simulink model "ResearchPaper3Fig3"  (R2015b)
settings: Solver=VariableStepAuto  StartTime=0.0  StopTime=10.0  RelTol=1e-3
libraries: xbsIndex_r4 x544, commfilt2 x1, commrandsrc3 x1, commdigbbndam3 x1
(part 1 of 4)
settings Model: Creator=barna  LastModifiedBy=barna

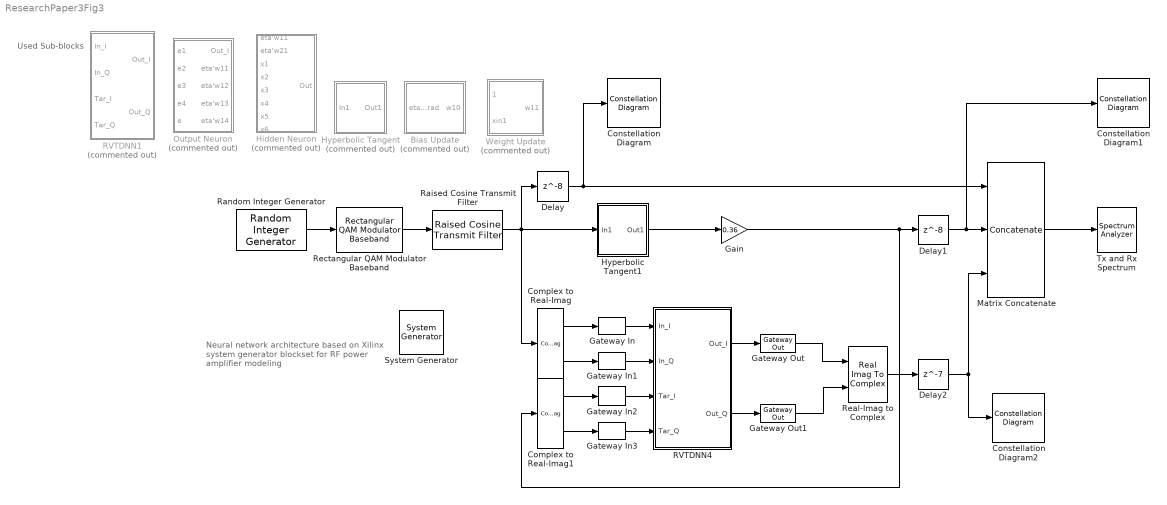
== system ResearchPaper3Fig3 ==
  note: Neural network architecture based on Xilinx system generator blockset for RF power amplifier modeling
  note: Used Sub-blocks
  " System Generator" : xbsIndex_r4/ System Generator  Tag=genX  xilinxfamily=kintex7  part=xc7k325t  speed=-3  package=fbg676  synthesis_tool=Vivado  clock_wrapper=Clock Enables  directory=./netlist  proj_type=Vivado  Synth_file=Vivado Synthesis Defaults  Impl_file=Vivado Implementation Defaults  testbench=off  simulink_period=1  sysclk_period=10  dcm_input_clock_period=10  incr_netlist=off  trim_vbits=Everywhere in SubSystem  dbl_ovrd=According to Block Masks  core_generation=According to Block Masks  run_coregen=off  deprecated_control=off  eval_field=0  block_type=sysgen
  Bias Update : Subsystem  Commented=on
  Complex to Real-Imag : ComplexToRealImag
  Complex to Real-Imag1 : ComplexToRealImag
  Constellation Diagram : ConstellationDiagram
  Constellation Diagram1 : ConstellationDiagram
  Constellation Diagram2 : ConstellationDiagram
  Delay : Delay  DelayLength=8  InitialCondition=0
  Delay1 : Delay  DelayLength=8  InitialCondition=0
  Delay2 : Delay  DelayLength=7  InitialCondition=0
  Gain : Gain  Gain=0.36
  Gateway In{,1..3} (4 alike) : xbsIndex_r4/Gateway In  gui_display_data_type=Fixed-point  arith_type="Signed  (2's comp)"  n_bits=16  bin_pt=14  preci_type=Single  exp_width=8  frac_width=24  rows=1  columns=1  quantization="Round  (unbiased: +/- Inf)"  overflow=Saturate  period=1  UseAsADC=off  ADCChannel='1'  interface=None  automatic_assignment=on  address_offset=hex2dec('00')  intf_name=''  intf_description=''  default_value=0  timing_constraint=None  locs_specified=off  LOCs={}  io_standard={}  inherit_from_input=off  hdl_port=on  dbl_ovrd=off  block_type=gatewayin
  Gateway Out : xbsIndex_r4/Gateway Out  inherit_from_input=off  hdl_port=on  rows=1  columns=1  UseAsDAC=off  DACChannel='1'  interface=None  automatic_assignment=on  address_offset=hex2dec('00')  intf_name=''  intf_description=''  timing_constraint=None  locs_specified=off  LOCs={}  io_standard={}  block_type=gatewayout
  Gateway Out1 : xbsIndex_r4/Gateway Out  inherit_from_input=off  hdl_port=on  rows=1  columns=1  UseAsDAC=off  DACChannel='1'  interface=None  automatic_assignment=on  address_offset=hex2dec('00')  intf_name=''  intf_description=''  timing_constraint=None  locs_specified=off  LOCs={}  io_standard={}  block_type=gatewayout
  Hidden Neuron : Subsystem  Commented=on
  Hyperbolic Tangent : Subsystem  Commented=on
  Hyperbolic Tangent1 : Subsystem
  Matrix Concatenate : Concatenate  NumInputs=3  Mode=Multidimensional array  ConcatenateDimension=2
  Output Neuron : Subsystem  Commented=on
  RVTDNN1 : Subsystem  Commented=on
  RVTDNN4 : Subsystem
  Raised Cosine Transmit Filter : commfilt2/Raised Cosine Transmit Filter  filtType=Normal  filtSpan=20  currentFiltSpan=20  D=(20)/2  R=0.2  sampMode=Mute  saveAsFlag=0  N=20  framing=Enforce single-rate processing  InputProcessing=Columns as channels (frame based)  checkGain=Normalized  filterGain=1  checkCoeff=off  variableName=rcTxFilt  launchFVT=on  roundingMode=Floor  overflowMode=off
  Random Integer Generator : commrandsrc3/Random Integer Generator  SetSize=8  SeedSource=Auto  Seed=0  SampleTime=1  SamplesPerFrame=1  OutputDataType=double  SimulateUsing=Interpreted execution
  Real-Imag to Complex : RealImagToComplex
  Rectangular QAM Modulator Baseband : commdigbbndam3/Rectangular QAM Modulator Baseband  M=16  InType=Integer  Enc=Gray  Mapping=[0:15]  PowType=Min. distance between symbols  MinDist=2  AvgPow=1  PeakPow=1  Ph=0  outDtype=double  outWordLen=16  outUDDataType=sfix(16)  outFracLenMode=Best precision  outFracLen=15
  Tx and Rx Spectrum : SpectrumAnalyzer
  Weight Update : Subsystem  Commented=on
  wires:
  Random Integer Generator/1 -> Rectangular QAM Modulator Baseband/1
  Rectangular QAM Modulator Baseband/1 -> Raised Cosine Transmit Filter/1
  Raised Cosine Transmit Filter/1 -> Hyperbolic Tangent1/1(In1), Complex to Real-Imag/1, Delay/1
  Complex to Real-Imag/1 -> Gateway In/1
  Complex to Real-Imag/2 -> Gateway In1/1
  Complex to Real-Imag1/1 -> Gateway In2/1
  Complex to Real-Imag1/2 -> Gateway In3/1
  Gateway Out/1 -> Real-Imag to Complex/1
  Gateway Out1/1 -> Real-Imag to Complex/2
  Gain/1 -> Complex to Real-Imag1/1, Delay1/1
  Real-Imag to Complex/1 -> Delay2/1
  Delay1/1 -> Constellation Diagram1/1, Matrix Concatenate/2
  Delay/1 -> Constellation Diagram/1, Matrix Concatenate/1
  Delay2/1 -> Matrix Concatenate/3, Constellation Diagram2/1
  Matrix Concatenate/1 -> Tx and Rx Spectrum/1
  Gateway In/1 -> RVTDNN4/1(In_I)
  Gateway In1/1 -> RVTDNN4/2(In_Q)
  Gateway In2/1 -> RVTDNN4/3(Tar_I)
  Gateway In3/1 -> RVTDNN4/4(Tar_Q)
  RVTDNN4/2(Out_Q) -> Gateway Out1/1
  RVTDNN4/1(Out_I) -> Gateway Out/1
  Hyperbolic Tangent1/1(Out1) -> Gain/1

== system ResearchPaper3Fig3/Bias Update ==
  eta'grad : Inport
  AddSub : xbsIndex_r4/AddSub  mode=Addition  use_carryin=off  use_carryout=off  en=off  latency=0  precision=Full  arith_type=Unsigned  n_bits=16  bin_pt=14  quantization=Truncate  overflow=Wrap  use_behavioral_HDL=off  hw_selection=Fabric  pipelined=off  dbl_ovrd=off  block_type=addsub
  Register : xbsIndex_r4/Register  init=0  rst=off  en=off  dbl_ovrd=off  block_type=register
  w10 : Outport
  wires:
  Register/1 -> w10/1, AddSub/2
  AddSub/1 -> Register/1
  eta'grad/1 -> AddSub/1

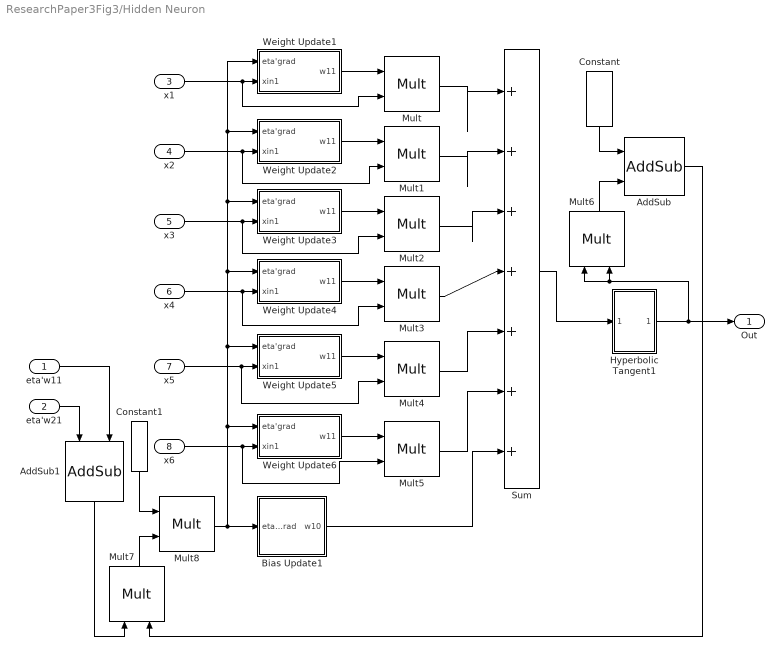
== system ResearchPaper3Fig3/Hidden Neuron ==
  eta'w11 : Inport
  eta'w21 : Inport  Port=2
  x1 : Inport  Port=3
  x2 : Inport  Port=4
  x3 : Inport  Port=5
  x4 : Inport  Port=6
  x5 : Inport  Port=7
  x6 : Inport  Port=8
  AddSub : xbsIndex_r4/AddSub  mode=Subtraction  use_carryin=off  use_carryout=off  en=off  latency=0  precision=Full  arith_type=Unsigned  n_bits=16  bin_pt=14  quantization=Truncate  overflow=Wrap  use_behavioral_HDL=off  hw_selection=Fabric  pipelined=off  dbl_ovrd=off  block_type=addsub
  AddSub1 : xbsIndex_r4/AddSub  mode=Addition  use_carryin=off  use_carryout=off  en=off  latency=0  precision=Full  arith_type=Unsigned  n_bits=16  bin_pt=14  quantization=Truncate  overflow=Wrap  use_behavioral_HDL=off  hw_selection=Fabric  pipelined=off  dbl_ovrd=off  block_type=addsub
  Bias Update1 : Subsystem
  Constant : xbsIndex_r4/Constant  const=1.0  gui_display_data_type=Fixed-point  arith_type=Signed (2's comp)  n_bits=16  bin_pt=14  preci_type=Single  exp_width=8  frac_width=24  explicit_period=off  period=1  equ=P=C  opselect=C  inp2=PCIN>>17  opr=+  inp1=P  carry=CIN  dbl_ovrd=off  block_type=constant
  Constant1 : xbsIndex_r4/Constant  const=0.1000000  gui_display_data_type=Fixed-point  arith_type=Signed (2's comp)  n_bits=32  bin_pt=24  preci_type=Single  exp_width=8  frac_width=24  explicit_period=off  period=1  equ=P=C  opselect=C  inp2=PCIN>>17  opr=+  inp1=P  carry=CIN  dbl_ovrd=off  block_type=constant
  Hyperbolic Tangent1 : Subsystem
  Mult{,1..8} (9 alike) : xbsIndex_r4/Mult  precision=Full  arith_type="Signed  (2's comp)"  n_bits=16  bin_pt=14  quantization=Truncate  overflow=Wrap  en=off  latency=0  use_behavioral_HDL=off  opt=Speed  use_embedded=on  optimum_pipeline=off  pipeline=on  dbl_ovrd=off  use_rpm=on  placement_style=Triangular  block_type=mult
  Sum : Sum  Inputs=|+++++++
  Weight Update1 : Subsystem
  Weight Update2 : Subsystem
  Weight Update3 : Subsystem
  Weight Update4 : Subsystem
  Weight Update5 : Subsystem
  Weight Update6 : Subsystem
  Out : Outport
  wires:
  Mult7/1 -> Mult8/2
  Sum/1 -> Hyperbolic Tangent1/1(In1)
  Bias Update1/1(w10) -> Sum/7
  Constant/1 -> AddSub/1
  Mult8/1 -> Weight Update6/1(eta'grad), Weight Update5/1(eta'grad), Weight Update4/1(eta'grad), Weight Update3/1(eta'grad), Weight Update2/1(eta'grad), Weight Update1/1(eta'grad), Bias Update1/1(eta'grad)
  Constant1/1 -> Mult8/1
  Mult6/1 -> AddSub/2
  eta'w11/1 -> AddSub1/2
  Hyperbolic Tangent1/1(Out1) -> Out/1, Mult6/1, Mult6/2
  AddSub1/1 -> Mult7/1
  AddSub/1 -> Mult7/2
  eta'w21/1 -> AddSub1/1
  Weight Update5/1(w11) -> Mult4/1
  x3/1 -> Mult2/2, Weight Update3/2(xin1)
  x5/1 -> Mult4/2, Weight Update5/2(xin1)
  Weight Update6/1(w11) -> Mult5/1
  Weight Update4/1(w11) -> Mult3/1
  x2/1 -> Mult1/2, Weight Update2/2(xin1)
  Weight Update1/1(w11) -> Mult/1
  Weight Update2/1(w11) -> Mult1/1
  Weight Update3/1(w11) -> Mult2/1
  x1/1 -> Mult/2, Weight Update1/2(xin1)
  x4/1 -> Mult3/2, Weight Update4/2(xin1)
  Mult1/1 -> Sum/2
  Mult4/1 -> Sum/5
  x6/1 -> Mult5/2, Weight Update6/2(xin1)
  Mult3/1 -> Sum/4
  Mult5/1 -> Sum/6
  Mult/1 -> Sum/1
  Mult2/1 -> Sum/3

== system ResearchPaper3Fig3/Hyperbolic Tangent ==
  In1 : Inport
  CMult : xbsIndex_r4/CMult  const=16380  gui_display_data_type=Fixed-point  const_n_bits=32  const_bin_pt=14  float_type=Single  exp_bits=8  fraction_bits=24  en=off  latency=0  precision=Full  arith_type="Signed  (2's comp)"  n_bits=16  bin_pt=14  quantization=Truncate  overflow=Wrap  use_behavioral_HDL=off  mem_type=Distributed RAM  pipeline=off  dbl_ovrd=off  block_type=cmult
  Constant : xbsIndex_r4/Constant  const=0.0  gui_display_data_type=Fixed-point  arith_type=Signed (2's comp)  n_bits=16  bin_pt=14  preci_type=Single  exp_width=8  frac_width=24  explicit_period=off  period=1  equ=P=C  opselect=C  inp2=PCIN>>17  opr=+  inp1=P  carry=CIN  dbl_ovrd=off  block_type=constant
  Delay1 : xbsIndex_r4/Delay  rst=off  infoeditControl=Selection of Reset will increase slice count due to use of real FFs and instead of SRLs  en=off  latency=1  reg_retiming=off  dbl_ovrd=off  block_type=delay
  Mux : xbsIndex_r4/Mux  inputs=2  en=off  latency=0  precision=Full  arith_type=Unsigned  n_bits=16  bin_pt=14  quantization=Truncate  overflow=Wrap  dbl_ovrd=off  block_type=mux
  Mux1 : xbsIndex_r4/Mux  inputs=2  en=off  latency=0  precision=Full  arith_type=Unsigned  n_bits=16  bin_pt=14  quantization=Truncate  overflow=Wrap  dbl_ovrd=off  block_type=mux
  Negate : xbsIndex_r4/Negate  precision=Full  arith_type=Unsigned  n_bits=16  bin_pt=14  quantization=Truncate  overflow=Wrap  en=off  latency=0  dbl_ovrd=off  block_type=negate
  Negate1 : xbsIndex_r4/Negate  precision=Full  arith_type=Unsigned  n_bits=16  bin_pt=14  quantization=Truncate  overflow=Wrap  en=off  latency=0  dbl_ovrd=off  block_type=negate
  ROM : xbsIndex_r4/ROM  depth=16  initVector=sin(pi*(0:15)/16)  distributed_mem=Block RAM  rst=off  init_reg=0  en=off  latency=1  gui_display_data_type=Fixed-point  arith_type="Signed  (2's comp)"  n_bits=16  bin_pt=14  preci_type=Single  exp_width=8  frac_width=24  optimize=Area  use_rpm=on  dbl_ovrd=off  block_type=sprom
  Relational : xbsIndex_r4/Relational  mode=a>b  op_type=Bool  en=off  latency=0  dbl_ovrd=off  block_type=relational
  Out1 : Outport
  wires:
  Delay1/1 -> Mux1/1
  Mux/1 -> CMult/1
  Mux1/1 -> Out1/1
  ROM/1 -> Negate1/1, Mux1/2
  Negate1/1 -> Mux1/3
  Relational/1 -> Delay1/1, Mux/1
  Constant/1 -> Relational/1
  In1/1 -> Negate/1, Relational/2, Mux/2
  Negate/1 -> Mux/3
  CMult/1 -> ROM/1

== system ResearchPaper3Fig3/Hyperbolic Tangent1 ==
  In1 : Inport
  CMult : xbsIndex_r4/CMult  const=16380  gui_display_data_type=Fixed-point  const_n_bits=32  const_bin_pt=14  float_type=Single  exp_bits=8  fraction_bits=24  en=off  latency=0  precision=Full  arith_type="Signed  (2's comp)"  n_bits=16  bin_pt=14  quantization=Truncate  overflow=Wrap  use_behavioral_HDL=off  mem_type=Distributed RAM  pipeline=off  dbl_ovrd=off  block_type=cmult
  Constant : xbsIndex_r4/Constant  const=0.0  gui_display_data_type=Fixed-point  arith_type=Signed (2's comp)  n_bits=16  bin_pt=14  preci_type=Single  exp_width=8  frac_width=24  explicit_period=off  period=1  equ=P=C  opselect=C  inp2=PCIN>>17  opr=+  inp1=P  carry=CIN  dbl_ovrd=off  block_type=constant
  Delay1 : xbsIndex_r4/Delay  rst=off  infoeditControl=Selection of Reset will increase slice count due to use of real FFs and instead of SRLs  en=off  latency=1  reg_retiming=off  dbl_ovrd=off  block_type=delay
  Mux : xbsIndex_r4/Mux  inputs=2  en=off  latency=0  precision=Full  arith_type=Unsigned  n_bits=16  bin_pt=14  quantization=Truncate  overflow=Wrap  dbl_ovrd=off  block_type=mux
  Mux1 : xbsIndex_r4/Mux  inputs=2  en=off  latency=0  precision=Full  arith_type=Unsigned  n_bits=16  bin_pt=14  quantization=Truncate  overflow=Wrap  dbl_ovrd=off  block_type=mux
  Negate : xbsIndex_r4/Negate  precision=Full  arith_type=Unsigned  n_bits=16  bin_pt=14  quantization=Truncate  overflow=Wrap  en=off  latency=0  dbl_ovrd=off  block_type=negate
  Negate1 : xbsIndex_r4/Negate  precision=Full  arith_type=Unsigned  n_bits=16  bin_pt=14  quantization=Truncate  overflow=Wrap  en=off  latency=0  dbl_ovrd=off  block_type=negate
  ROM : xbsIndex_r4/ROM  depth=16  initVector=sin(pi*(0:15)/16)  distributed_mem=Block RAM  rst=off  init_reg=0  en=off  latency=1  gui_display_data_type=Fixed-point  arith_type="Signed  (2's comp)"  n_bits=16  bin_pt=14  preci_type=Single  exp_width=8  frac_width=24  optimize=Area  use_rpm=on  dbl_ovrd=off  block_type=sprom
  Relational : xbsIndex_r4/Relational  mode=a>b  op_type=Bool  en=off  latency=0  dbl_ovrd=off  block_type=relational
  Out1 : Outport
  wires:
  Delay1/1 -> Mux1/1
  Mux/1 -> CMult/1
  Mux1/1 -> Out1/1
  ROM/1 -> Negate1/1, Mux1/2
  Negate1/1 -> Mux1/3
  Relational/1 -> Delay1/1, Mux/1
  Constant/1 -> Relational/1
  In1/1 -> Negate/1, Relational/2, Mux/2
  Negate/1 -> Mux/3
  CMult/1 -> ROM/1

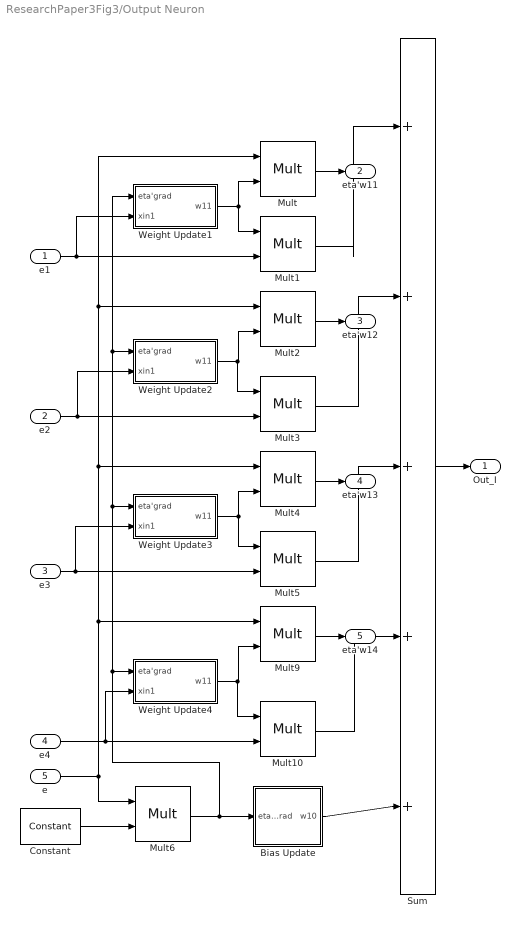
== system ResearchPaper3Fig3/Output Neuron ==
  e1 : Inport
  e2 : Inport  Port=2
  e3 : Inport  Port=3
  e4 : Inport  Port=4
  e : Inport  Port=5
  Bias Update : Subsystem
  Constant : xbsIndex_r4/Constant  const=16972656  gui_display_data_type=Fixed-point  arith_type=Signed (2's comp)  n_bits=64  bin_pt=14  preci_type=Single  exp_width=8  frac_width=24  explicit_period=off  period=1  equ=P=C  opselect=C  inp2=PCIN>>17  opr=+  inp1=P  carry=CIN  dbl_ovrd=off  block_type=constant
  Mult{,1..6,9..10} (9 alike) : xbsIndex_r4/Mult  precision=Full  arith_type="Signed  (2's comp)"  n_bits=16  bin_pt=14  quantization=Truncate  overflow=Wrap  en=off  latency=0  use_behavioral_HDL=off  opt=Speed  use_embedded=on  optimum_pipeline=off  pipeline=on  dbl_ovrd=off  use_rpm=on  placement_style=Triangular  block_type=mult
  Sum : Sum  Inputs=|+++++
  Weight Update1 : Subsystem
  Weight Update2 : Subsystem
  Weight Update3 : Subsystem
  Weight Update4 : Subsystem
  Out_I : Outport
  eta'w11 : Outport  Port=2
  eta'w12 : Outport  Port=3
  eta'w13 : Outport  Port=4
  eta'w14 : Outport  Port=5
  wires:
  e3/1 -> Weight Update3/2(xin1), Mult5/2
  e2/1 -> Weight Update2/2(xin1), Mult3/2
  e1/1 -> Weight Update1/2(xin1), Mult1/2
  e4/1 -> Weight Update4/2(xin1), Mult10/2
  Weight Update1/1(w11) -> Mult1/1, Mult/2
  Weight Update2/1(w11) -> Mult3/1, Mult2/2
  Weight Update3/1(w11) -> Mult5/1, Mult4/2
  Weight Update4/1(w11) -> Mult10/1, Mult9/2
  Mult/1 -> eta'w11/1
  Mult2/1 -> eta'w12/1
  Mult4/1 -> eta'w13/1
  Mult9/1 -> eta'w14/1
  Mult1/1 -> Sum/1
  Mult3/1 -> Sum/2
  Mult5/1 -> Sum/3
  Mult10/1 -> Sum/4
  Bias Update/1(w10) -> Sum/5
  Mult6/1 -> Weight Update4/1(eta'grad), Weight Update3/1(eta'grad), Weight Update2/1(eta'grad), Weight Update1/1(eta'grad), Bias Update/1(eta'grad)
  Constant/1 -> Mult6/2
  e/1 -> Mult4/1, Mult2/1, Mult/1, Mult9/1, Mult6/1
  Sum/1 -> Out_I/1

== system ResearchPaper3Fig3/RVTDNN1 ==
  In_I : Inport
  In_Q : Inport  Port=2
  Tar_I : Inport  Port=3
  Tar_Q : Inport  Port=4
  AddSub : xbsIndex_r4/AddSub  mode=Subtraction  use_carryin=off  use_carryout=off  en=off  latency=1  precision=Full  arith_type=Unsigned  n_bits=16  bin_pt=14  quantization=Truncate  overflow=Wrap  use_behavioral_HDL=off  hw_selection=Fabric  pipelined=off  dbl_ovrd=off  block_type=addsub
  AddSub1 : xbsIndex_r4/AddSub  mode=Subtraction  use_carryin=off  use_carryout=off  en=off  latency=1  precision=Full  arith_type=Unsigned  n_bits=16  bin_pt=14  quantization=Truncate  overflow=Wrap  use_behavioral_HDL=off  hw_selection=Fabric  pipelined=off  dbl_ovrd=off  block_type=addsub
  Delay{3..8} (6 alike) : xbsIndex_r4/Delay  rst=off  infoeditControl=Selection of Reset will increase slice count due to use of real FFs and instead of SRLs  en=off  latency=1  reg_retiming=off  dbl_ovrd=off  block_type=delay
  Hidden Neuron1 : Subsystem
  Hidden Neuron2 : Subsystem
  Hidden Neuron3 : Subsystem
  Hidden Neuron4 : Subsystem
  Output Neuron1 : Subsystem
  Output Neuron2 : Subsystem
  Out_I : Outport
  Out_Q : Outport  Port=2
  wires:
  Output Neuron2/1(Out_I) -> Out_Q/1, AddSub1/2
  Delay7/1 -> AddSub/1
  Output Neuron1/2(eta'w11) -> Hidden Neuron1/1(eta'w11)
  Delay8/1 -> AddSub1/1
  In_Q/1 -> Hidden Neuron3/6(x4), Hidden Neuron4/6(x4), Hidden Neuron1/6(x4), Hidden Neuron2/6(x4), Delay5/1
  Delay5/1 -> Hidden Neuron1/7(x5), Hidden Neuron2/7(x5), Hidden Neuron3/7(x5), Hidden Neuron4/7(x5), Delay6/1
  Delay3/1 -> Hidden Neuron2/4(x2), Hidden Neuron3/4(x2), Hidden Neuron4/4(x2), Hidden Neuron1/4(x2), Delay4/1
  Output Neuron2/3(eta'w12) -> Hidden Neuron2/2(eta'w21)
  Output Neuron2/4(eta'w13) -> Hidden Neuron3/2(eta'w21)
  AddSub/1 -> Output Neuron1/5(e)
  In_I/1 -> Hidden Neuron1/3(x1), Hidden Neuron2/3(x1), Hidden Neuron3/3(x1), Hidden Neuron4/3(x1), Delay3/1
  Output Neuron2/5(eta'w14) -> Hidden Neuron4/2(eta'w21)
  Hidden Neuron1/1(Out) -> Output Neuron2/1(e1), Output Neuron1/1(e1)
  Hidden Neuron4/1(Out) -> Output Neuron2/4(e4), Output Neuron1/4(e4)
  Hidden Neuron3/1(Out) -> Output Neuron2/3(e3), Output Neuron1/3(e3)
  Hidden Neuron2/1(Out) -> Output Neuron2/2(e2), Output Neuron1/2(e2)
  Output Neuron1/3(eta'w12) -> Hidden Neuron2/1(eta'w11)
  Output Neuron1/4(eta'w13) -> Hidden Neuron3/1(eta'w11)
  Output Neuron1/5(eta'w14) -> Hidden Neuron4/1(eta'w11)
  Output Neuron2/2(eta'w11) -> Hidden Neuron1/2(eta'w21)
  Delay6/1 -> Hidden Neuron1/8(x6), Hidden Neuron2/8(x6), Hidden Neuron3/8(x6), Hidden Neuron4/8(x6)
  Delay4/1 -> Hidden Neuron3/5(x3), Hidden Neuron4/5(x3), Hidden Neuron1/5(x3), Hidden Neuron2/5(x3)
  Tar_Q/1 -> Delay8/1
  Tar_I/1 -> Delay7/1
  AddSub1/1 -> Output Neuron2/5(e)
  Output Neuron1/1(Out_I) -> Out_I/1, AddSub/2

== system ResearchPaper3Fig3/RVTDNN4 ==
  In_I : Inport
  In_Q : Inport  Port=2
  Tar_I : Inport  Port=3
  Tar_Q : Inport  Port=4
  AddSub : xbsIndex_r4/AddSub  mode=Subtraction  use_carryin=off  use_carryout=off  en=off  latency=0  precision=Full  arith_type=Unsigned  n_bits=16  bin_pt=14  quantization=Truncate  overflow=Wrap  use_behavioral_HDL=off  hw_selection=Fabric  pipelined=off  dbl_ovrd=off  block_type=addsub
  AddSub1 : xbsIndex_r4/AddSub  mode=Subtraction  use_carryin=off  use_carryout=off  en=off  latency=0  precision=Full  arith_type=Unsigned  n_bits=16  bin_pt=14  quantization=Truncate  overflow=Wrap  use_behavioral_HDL=off  hw_selection=Fabric  pipelined=off  dbl_ovrd=off  block_type=addsub
  Delay{3..8} (6 alike) : xbsIndex_r4/Delay  rst=off  infoeditControl=Selection of Reset will increase slice count due to use of real FFs and instead of SRLs  en=off  latency=1  reg_retiming=off  dbl_ovrd=off  block_type=delay
  Hidden Neuron1 : Subsystem
  Hidden Neuron2 : Subsystem
  Hidden Neuron3 : Subsystem
  Hidden Neuron4 : Subsystem
  Output Neuron1 : Subsystem
  Output Neuron2 : Subsystem
  Out_I : Outport
  Out_Q : Outport  Port=2
  wires:
  Output Neuron2/1(Out_I) -> Out_Q/1, AddSub1/2
  Delay7/1 -> AddSub/1
  Output Neuron1/2(eta'w11) -> Hidden Neuron1/1(eta'w11)
  Delay8/1 -> AddSub1/1
  In_Q/1 -> Hidden Neuron3/6(x4), Hidden Neuron4/6(x4), Hidden Neuron1/6(x4), Hidden Neuron2/6(x4), Delay5/1
  Delay5/1 -> Hidden Neuron1/7(x5), Hidden Neuron2/7(x5), Hidden Neuron3/7(x5), Hidden Neuron4/7(x5), Delay6/1
  Delay3/1 -> Hidden Neuron2/4(x2), Hidden Neuron3/4(x2), Hidden Neuron4/4(x2), Hidden Neuron1/4(x2), Delay4/1
  Output Neuron2/3(eta'w12) -> Hidden Neuron2/2(eta'w21)
  Output Neuron2/4(eta'w13) -> Hidden Neuron3/2(eta'w21)
  AddSub/1 -> Output Neuron1/5(e)
  In_I/1 -> Hidden Neuron1/3(x1), Hidden Neuron2/3(x1), Hidden Neuron3/3(x1), Hidden Neuron4/3(x1), Delay3/1
  Output Neuron2/5(eta'w14) -> Hidden Neuron4/2(eta'w21)
  Hidden Neuron1/1(Out) -> Output Neuron2/1(e1), Output Neuron1/1(e1)
  Hidden Neuron4/1(Out) -> Output Neuron2/4(e4), Output Neuron1/4(e4)
  Hidden Neuron3/1(Out) -> Output Neuron2/3(e3), Output Neuron1/3(e3)
  Hidden Neuron2/1(Out) -> Output Neuron2/2(e2), Output Neuron1/2(e2)
  Output Neuron1/3(eta'w12) -> Hidden Neuron2/1(eta'w11)
  Output Neuron1/4(eta'w13) -> Hidden Neuron3/1(eta'w11)
  Output Neuron1/5(eta'w14) -> Hidden Neuron4/1(eta'w11)
  Output Neuron2/2(eta'w11) -> Hidden Neuron1/2(eta'w21)
  Delay6/1 -> Hidden Neuron1/8(x6), Hidden Neuron2/8(x6), Hidden Neuron3/8(x6), Hidden Neuron4/8(x6)
  Delay4/1 -> Hidden Neuron3/5(x3), Hidden Neuron4/5(x3), Hidden Neuron1/5(x3), Hidden Neuron2/5(x3)
  Tar_Q/1 -> Delay8/1
  Tar_I/1 -> Delay7/1
  AddSub1/1 -> Output Neuron2/5(e)
  Output Neuron1/1(Out_I) -> Out_I/1, AddSub/2

== system ResearchPaper3Fig3/Weight Update ==
  eta'grad : Inport
  xin1 : Inport  Port=2
  AddSub : xbsIndex_r4/AddSub  mode=Addition  use_carryin=off  use_carryout=off  en=off  latency=0  precision=Full  arith_type=Unsigned  n_bits=16  bin_pt=14  quantization=Truncate  overflow=Wrap  use_behavioral_HDL=off  hw_selection=Fabric  pipelined=off  dbl_ovrd=off  block_type=addsub
  Mult : xbsIndex_r4/Mult  precision=Full  arith_type="Signed  (2's comp)"  n_bits=16  bin_pt=14  quantization=Truncate  overflow=Wrap  en=off  latency=0  use_behavioral_HDL=off  opt=Speed  use_embedded=on  optimum_pipeline=off  pipeline=on  dbl_ovrd=off  use_rpm=on  placement_style=Triangular  block_type=mult
  Register : xbsIndex_r4/Register  init=0  rst=off  en=off  dbl_ovrd=off  block_type=register
  w11 : Outport
  wires:
  Mult/1 -> AddSub/1
  Register/1 -> w11/1, AddSub/2
  AddSub/1 -> Register/1
  eta'grad/1 -> Mult/1
  xin1/1 -> Mult/2

== system ResearchPaper3Fig3/Hidden Neuron/Bias Update1 ==
  eta'grad : Inport
  AddSub : xbsIndex_r4/AddSub  mode=Addition  use_carryin=off  use_carryout=off  en=off  latency=0  precision=Full  arith_type=Unsigned  n_bits=16  bin_pt=14  quantization=Truncate  overflow=Wrap  use_behavioral_HDL=off  hw_selection=Fabric  pipelined=off  dbl_ovrd=off  block_type=addsub
  Register : xbsIndex_r4/Register  init=0  rst=off  en=off  dbl_ovrd=off  block_type=register
  w10 : Outport
  wires:
  Register/1 -> w10/1, AddSub/2
  AddSub/1 -> Register/1
  eta'grad/1 -> AddSub/1

== system ResearchPaper3Fig3/Hidden Neuron/Hyperbolic Tangent1 ==
  In1 : Inport
  CMult : xbsIndex_r4/CMult  const=16380  gui_display_data_type=Fixed-point  const_n_bits=32  const_bin_pt=14  float_type=Single  exp_bits=8  fraction_bits=24  en=off  latency=0  precision=Full  arith_type="Signed  (2's comp)"  n_bits=16  bin_pt=14  quantization=Truncate  overflow=Wrap  use_behavioral_HDL=off  mem_type=Distributed RAM  pipeline=off  dbl_ovrd=off  block_type=cmult
  Constant : xbsIndex_r4/Constant  const=0.0  gui_display_data_type=Fixed-point  arith_type=Signed (2's comp)  n_bits=16  bin_pt=14  preci_type=Single  exp_width=8  frac_width=24  explicit_period=off  period=1  equ=P=C  opselect=C  inp2=PCIN>>17  opr=+  inp1=P  carry=CIN  dbl_ovrd=off  block_type=constant
  Delay1 : xbsIndex_r4/Delay  rst=off  infoeditControl=Selection of Reset will increase slice count due to use of real FFs and instead of SRLs  en=off  latency=1  reg_retiming=off  dbl_ovrd=off  block_type=delay
  Mux : xbsIndex_r4/Mux  inputs=2  en=off  latency=0  precision=Full  arith_type=Unsigned  n_bits=16  bin_pt=14  quantization=Truncate  overflow=Wrap  dbl_ovrd=off  block_type=mux
  Mux1 : xbsIndex_r4/Mux  inputs=2  en=off  latency=0  precision=Full  arith_type=Unsigned  n_bits=16  bin_pt=14  quantization=Truncate  overflow=Wrap  dbl_ovrd=off  block_type=mux
  Negate : xbsIndex_r4/Negate  precision=Full  arith_type=Unsigned  n_bits=16  bin_pt=14  quantization=Truncate  overflow=Wrap  en=off  latency=0  dbl_ovrd=off  block_type=negate
  Negate1 : xbsIndex_r4/Negate  precision=Full  arith_type=Unsigned  n_bits=16  bin_pt=14  quantization=Truncate  overflow=Wrap  en=off  latency=0  dbl_ovrd=off  block_type=negate
  ROM : xbsIndex_r4/ROM  depth=16  initVector=sin(pi*(0:15)/16)  distributed_mem=Block RAM  rst=off  init_reg=0  en=off  latency=1  gui_display_data_type=Fixed-point  arith_type="Signed  (2's comp)"  n_bits=16  bin_pt=14  preci_type=Single  exp_width=8  frac_width=24  optimize=Area  use_rpm=on  dbl_ovrd=off  block_type=sprom
  Relational : xbsIndex_r4/Relational  mode=a>b  op_type=Bool  en=off  latency=0  dbl_ovrd=off  block_type=relational
  Out1 : Outport
  wires:
  Delay1/1 -> Mux1/1
  Mux/1 -> CMult/1
  Mux1/1 -> Out1/1
  ROM/1 -> Negate1/1, Mux1/2
  Negate1/1 -> Mux1/3
  Relational/1 -> Delay1/1, Mux/1
  Constant/1 -> Relational/1
  In1/1 -> Negate/1, Relational/2, Mux/2
  Negate/1 -> Mux/3
  CMult/1 -> ROM/1

== system ResearchPaper3Fig3/Hidden Neuron/Weight Update1 ==
  eta'grad : Inport
  xin1 : Inport  Port=2
  AddSub : xbsIndex_r4/AddSub  mode=Addition  use_carryin=off  use_carryout=off  en=off  latency=0  precision=Full  arith_type=Unsigned  n_bits=16  bin_pt=14  quantization=Truncate  overflow=Wrap  use_behavioral_HDL=off  hw_selection=Fabric  pipelined=off  dbl_ovrd=off  block_type=addsub
  Mult : xbsIndex_r4/Mult  precision=Full  arith_type="Signed  (2's comp)"  n_bits=16  bin_pt=14  quantization=Truncate  overflow=Wrap  en=off  latency=0  use_behavioral_HDL=off  opt=Speed  use_embedded=on  optimum_pipeline=off  pipeline=on  dbl_ovrd=off  use_rpm=on  placement_style=Triangular  block_type=mult
  Register : xbsIndex_r4/Register  init=0  rst=off  en=off  dbl_ovrd=off  block_type=register
  w11 : Outport
  wires:
  Mult/1 -> AddSub/1
  Register/1 -> w11/1, AddSub/2
  AddSub/1 -> Register/1
  eta'grad/1 -> Mult/1
  xin1/1 -> Mult/2

== system ResearchPaper3Fig3/Hidden Neuron/Weight Update2 ==
  eta'grad : Inport
  xin1 : Inport  Port=2
  AddSub : xbsIndex_r4/AddSub  mode=Addition  use_carryin=off  use_carryout=off  en=off  latency=0  precision=Full  arith_type=Unsigned  n_bits=16  bin_pt=14  quantization=Truncate  overflow=Wrap  use_behavioral_HDL=off  hw_selection=Fabric  pipelined=off  dbl_ovrd=off  block_type=addsub
  Mult : xbsIndex_r4/Mult  precision=Full  arith_type="Signed  (2's comp)"  n_bits=16  bin_pt=14  quantization=Truncate  overflow=Wrap  en=off  latency=0  use_behavioral_HDL=off  opt=Speed  use_embedded=on  optimum_pipeline=off  pipeline=on  dbl_ovrd=off  use_rpm=on  placement_style=Triangular  block_type=mult
  Register : xbsIndex_r4/Register  init=0  rst=off  en=off  dbl_ovrd=off  block_type=register
  w11 : Outport
  wires:
  Mult/1 -> AddSub/1
  Register/1 -> w11/1, AddSub/2
  AddSub/1 -> Register/1
  eta'grad/1 -> Mult/1
  xin1/1 -> Mult/2

== system ResearchPaper3Fig3/Hidden Neuron/Weight Update3 ==
  eta'grad : Inport
  xin1 : Inport  Port=2
  AddSub : xbsIndex_r4/AddSub  mode=Addition  use_carryin=off  use_carryout=off  en=off  latency=0  precision=Full  arith_type=Unsigned  n_bits=16  bin_pt=14  quantization=Truncate  overflow=Wrap  use_behavioral_HDL=off  hw_selection=Fabric  pipelined=off  dbl_ovrd=off  block_type=addsub
  Mult : xbsIndex_r4/Mult  precision=Full  arith_type="Signed  (2's comp)"  n_bits=16  bin_pt=14  quantization=Truncate  overflow=Wrap  en=off  latency=0  use_behavioral_HDL=off  opt=Speed  use_embedded=on  optimum_pipeline=off  pipeline=on  dbl_ovrd=off  use_rpm=on  placement_style=Triangular  block_type=mult
  Register : xbsIndex_r4/Register  init=0  rst=off  en=off  dbl_ovrd=off  block_type=register
  w11 : Outport
  wires:
  Mult/1 -> AddSub/1
  Register/1 -> w11/1, AddSub/2
  AddSub/1 -> Register/1
  eta'grad/1 -> Mult/1
  xin1/1 -> Mult/2

== system ResearchPaper3Fig3/Hidden Neuron/Weight Update4 ==
  eta'grad : Inport
  xin1 : Inport  Port=2
  AddSub : xbsIndex_r4/AddSub  mode=Addition  use_carryin=off  use_carryout=off  en=off  latency=0  precision=Full  arith_type=Unsigned  n_bits=16  bin_pt=14  quantization=Truncate  overflow=Wrap  use_behavioral_HDL=off  hw_selection=Fabric  pipelined=off  dbl_ovrd=off  block_type=addsub
  Mult : xbsIndex_r4/Mult  precision=Full  arith_type="Signed  (2's comp)"  n_bits=16  bin_pt=14  quantization=Truncate  overflow=Wrap  en=off  latency=0  use_behavioral_HDL=off  opt=Speed  use_embedded=on  optimum_pipeline=off  pipeline=on  dbl_ovrd=off  use_rpm=on  placement_style=Triangular  block_type=mult
  Register : xbsIndex_r4/Register  init=0  rst=off  en=off  dbl_ovrd=off  block_type=register
  w11 : Outport
  wires:
  Mult/1 -> AddSub/1
  Register/1 -> w11/1, AddSub/2
  AddSub/1 -> Register/1
  eta'grad/1 -> Mult/1
  xin1/1 -> Mult/2

== system ResearchPaper3Fig3/Hidden Neuron/Weight Update5 ==
  eta'grad : Inport
  xin1 : Inport  Port=2
  AddSub : xbsIndex_r4/AddSub  mode=Addition  use_carryin=off  use_carryout=off  en=off  latency=0  precision=Full  arith_type=Unsigned  n_bits=16  bin_pt=14  quantization=Truncate  overflow=Wrap  use_behavioral_HDL=off  hw_selection=Fabric  pipelined=off  dbl_ovrd=off  block_type=addsub
  Mult : xbsIndex_r4/Mult  precision=Full  arith_type="Signed  (2's comp)"  n_bits=16  bin_pt=14  quantization=Truncate  overflow=Wrap  en=off  latency=0  use_behavioral_HDL=off  opt=Speed  use_embedded=on  optimum_pipeline=off  pipeline=on  dbl_ovrd=off  use_rpm=on  placement_style=Triangular  block_type=mult
  Register : xbsIndex_r4/Register  init=0  rst=off  en=off  dbl_ovrd=off  block_type=register
  w11 : Outport
  wires:
  Mult/1 -> AddSub/1
  Register/1 -> w11/1, AddSub/2
  AddSub/1 -> Register/1
  eta'grad/1 -> Mult/1
  xin1/1 -> Mult/2

== system ResearchPaper3Fig3/Hidden Neuron/Weight Update6 ==
  eta'grad : Inport
  xin1 : Inport  Port=2
  AddSub : xbsIndex_r4/AddSub  mode=Addition  use_carryin=off  use_carryout=off  en=off  latency=0  precision=Full  arith_type=Unsigned  n_bits=16  bin_pt=14  quantization=Truncate  overflow=Wrap  use_behavioral_HDL=off  hw_selection=Fabric  pipelined=off  dbl_ovrd=off  block_type=addsub
  Mult : xbsIndex_r4/Mult  precision=Full  arith_type="Signed  (2's comp)"  n_bits=16  bin_pt=14  quantization=Truncate  overflow=Wrap  en=off  latency=0  use_behavioral_HDL=off  opt=Speed  use_embedded=on  optimum_pipeline=off  pipeline=on  dbl_ovrd=off  use_rpm=on  placement_style=Triangular  block_type=mult
  Register : xbsIndex_r4/Register  init=0  rst=off  en=off  dbl_ovrd=off  block_type=register
  w11 : Outport
  wires:
  Mult/1 -> AddSub/1
  Register/1 -> w11/1, AddSub/2
  AddSub/1 -> Register/1
  eta'grad/1 -> Mult/1
  xin1/1 -> Mult/2

== system ResearchPaper3Fig3/Output Neuron/Bias Update ==
  eta'grad : Inport
  AddSub : xbsIndex_r4/AddSub  mode=Addition  use_carryin=off  use_carryout=off  en=off  latency=0  precision=Full  arith_type=Unsigned  n_bits=16  bin_pt=14  quantization=Truncate  overflow=Wrap  use_behavioral_HDL=off  hw_selection=Fabric  pipelined=off  dbl_ovrd=off  block_type=addsub
  Register : xbsIndex_r4/Register  init=0  rst=off  en=off  dbl_ovrd=off  block_type=register
  w10 : Outport
  wires:
  Register/1 -> w10/1, AddSub/2
  AddSub/1 -> Register/1
  eta'grad/1 -> AddSub/1

== system ResearchPaper3Fig3/Output Neuron/Weight Update1 ==
  eta'grad : Inport
  xin1 : Inport  Port=2
  AddSub : xbsIndex_r4/AddSub  mode=Addition  use_carryin=off  use_carryout=off  en=off  latency=0  precision=Full  arith_type=Unsigned  n_bits=16  bin_pt=14  quantization=Truncate  overflow=Wrap  use_behavioral_HDL=off  hw_selection=Fabric  pipelined=off  dbl_ovrd=off  block_type=addsub
  Mult : xbsIndex_r4/Mult  precision=Full  arith_type="Signed  (2's comp)"  n_bits=16  bin_pt=14  quantization=Truncate  overflow=Wrap  en=off  latency=0  use_behavioral_HDL=off  opt=Speed  use_embedded=on  optimum_pipeline=off  pipeline=on  dbl_ovrd=off  use_rpm=on  placement_style=Triangular  block_type=mult
  Register : xbsIndex_r4/Register  init=0  rst=off  en=off  dbl_ovrd=off  block_type=register
  w11 : Outport
  wires:
  Mult/1 -> AddSub/1
  Register/1 -> w11/1, AddSub/2
  AddSub/1 -> Register/1
  eta'grad/1 -> Mult/1
  xin1/1 -> Mult/2

== system ResearchPaper3Fig3/Output Neuron/Weight Update2 ==
  eta'grad : Inport
  xin1 : Inport  Port=2
  AddSub : xbsIndex_r4/AddSub  mode=Addition  use_carryin=off  use_carryout=off  en=off  latency=0  precision=Full  arith_type=Unsigned  n_bits=16  bin_pt=14  quantization=Truncate  overflow=Wrap  use_behavioral_HDL=off  hw_selection=Fabric  pipelined=off  dbl_ovrd=off  block_type=addsub
  Mult : xbsIndex_r4/Mult  precision=Full  arith_type="Signed  (2's comp)"  n_bits=16  bin_pt=14  quantization=Truncate  overflow=Wrap  en=off  latency=0  use_behavioral_HDL=off  opt=Speed  use_embedded=on  optimum_pipeline=off  pipeline=on  dbl_ovrd=off  use_rpm=on  placement_style=Triangular  block_type=mult
  Register : xbsIndex_r4/Register  init=0  rst=off  en=off  dbl_ovrd=off  block_type=register
  w11 : Outport
  wires:
  Mult/1 -> AddSub/1
  Register/1 -> w11/1, AddSub/2
  AddSub/1 -> Register/1
  eta'grad/1 -> Mult/1
  xin1/1 -> Mult/2

== system ResearchPaper3Fig3/Output Neuron/Weight Update3 ==
  eta'grad : Inport
  xin1 : Inport  Port=2
  AddSub : xbsIndex_r4/AddSub  mode=Addition  use_carryin=off  use_carryout=off  en=off  latency=0  precision=Full  arith_type=Unsigned  n_bits=16  bin_pt=14  quantization=Truncate  overflow=Wrap  use_behavioral_HDL=off  hw_selection=Fabric  pipelined=off  dbl_ovrd=off  block_type=addsub
  Mult : xbsIndex_r4/Mult  precision=Full  arith_type="Signed  (2's comp)"  n_bits=16  bin_pt=14  quantization=Truncate  overflow=Wrap  en=off  latency=0  use_behavioral_HDL=off  opt=Speed  use_embedded=on  optimum_pipeline=off  pipeline=on  dbl_ovrd=off  use_rpm=on  placement_style=Triangular  block_type=mult
  Register : xbsIndex_r4/Register  init=0  rst=off  en=off  dbl_ovrd=off  block_type=register
  w11 : Outport
  wires:
  Mult/1 -> AddSub/1
  Register/1 -> w11/1, AddSub/2
  AddSub/1 -> Register/1
  eta'grad/1 -> Mult/1
  xin1/1 -> Mult/2

== system ResearchPaper3Fig3/Output Neuron/Weight Update4 ==
  eta'grad : Inport
  xin1 : Inport  Port=2
  AddSub : xbsIndex_r4/AddSub  mode=Addition  use_carryin=off  use_carryout=off  en=off  latency=0  precision=Full  arith_type=Unsigned  n_bits=16  bin_pt=14  quantization=Truncate  overflow=Wrap  use_behavioral_HDL=off  hw_selection=Fabric  pipelined=off  dbl_ovrd=off  block_type=addsub
  Mult : xbsIndex_r4/Mult  precision=Full  arith_type="Signed  (2's comp)"  n_bits=16  bin_pt=14  quantization=Truncate  overflow=Wrap  en=off  latency=0  use_behavioral_HDL=off  opt=Speed  use_embedded=on  optimum_pipeline=off  pipeline=on  dbl_ovrd=off  use_rpm=on  placement_style=Triangular  block_type=mult
  Register : xbsIndex_r4/Register  init=0  rst=off  en=off  dbl_ovrd=off  block_type=register
  w11 : Outport
  wires:
  Mult/1 -> AddSub/1
  Register/1 -> w11/1, AddSub/2
  AddSub/1 -> Register/1
  eta'grad/1 -> Mult/1
  xin1/1 -> Mult/2

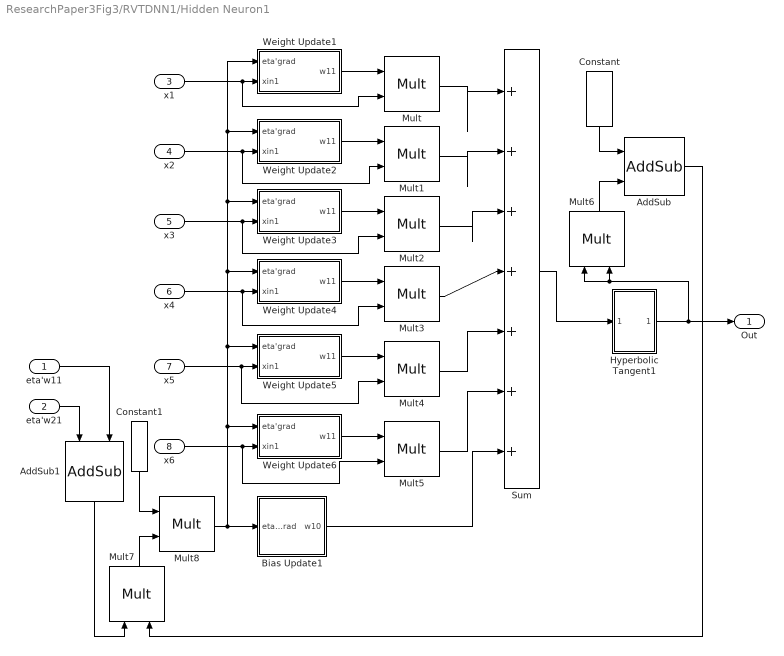
== system ResearchPaper3Fig3/RVTDNN1/Hidden Neuron1 ==
  eta'w11 : Inport
  eta'w21 : Inport  Port=2
  x1 : Inport  Port=3
  x2 : Inport  Port=4
  x3 : Inport  Port=5
  x4 : Inport  Port=6
  x5 : Inport  Port=7
  x6 : Inport  Port=8
  AddSub : xbsIndex_r4/AddSub  mode=Subtraction  use_carryin=off  use_carryout=off  en=off  latency=0  precision=Full  arith_type=Unsigned  n_bits=16  bin_pt=14  quantization=Truncate  overflow=Wrap  use_behavioral_HDL=off  hw_selection=Fabric  pipelined=off  dbl_ovrd=off  block_type=addsub
  AddSub1 : xbsIndex_r4/AddSub  mode=Addition  use_carryin=off  use_carryout=off  en=off  latency=0  precision=Full  arith_type=Unsigned  n_bits=16  bin_pt=14  quantization=Truncate  overflow=Wrap  use_behavioral_HDL=off  hw_selection=Fabric  pipelined=off  dbl_ovrd=off  block_type=addsub
  Bias Update1 : Subsystem
  Constant : xbsIndex_r4/Constant  const=1.0  gui_display_data_type=Fixed-point  arith_type=Signed (2's comp)  n_bits=16  bin_pt=14  preci_type=Single  exp_width=8  frac_width=24  explicit_period=off  period=1  equ=P=C  opselect=C  inp2=PCIN>>17  opr=+  inp1=P  carry=CIN  dbl_ovrd=off  block_type=constant
  Constant1 : xbsIndex_r4/Constant  const=0.1000000  gui_display_data_type=Fixed-point  arith_type=Signed (2's comp)  n_bits=32  bin_pt=24  preci_type=Single  exp_width=8  frac_width=24  explicit_period=off  period=1  equ=P=C  opselect=C  inp2=PCIN>>17  opr=+  inp1=P  carry=CIN  dbl_ovrd=off  block_type=constant
  Hyperbolic Tangent1 : Subsystem
  Mult{,1..8} (9 alike) : xbsIndex_r4/Mult  precision=Full  arith_type="Signed  (2's comp)"  n_bits=16  bin_pt=14  quantization=Truncate  overflow=Wrap  en=off  latency=0  use_behavioral_HDL=off  opt=Speed  use_embedded=on  optimum_pipeline=off  pipeline=on  dbl_ovrd=off  use_rpm=on  placement_style=Triangular  block_type=mult
  Sum : Sum  Inputs=|+++++++
  Weight Update1 : Subsystem
  Weight Update2 : Subsystem
  Weight Update3 : Subsystem
  Weight Update4 : Subsystem
  Weight Update5 : Subsystem
  Weight Update6 : Subsystem
  Out : Outport
  wires:
  Mult7/1 -> Mult8/2
  Sum/1 -> Hyperbolic Tangent1/1(In1)
  Bias Update1/1(w10) -> Sum/7
  Constant/1 -> AddSub/1
  Mult8/1 -> Weight Update6/1(eta'grad), Weight Update5/1(eta'grad), Weight Update4/1(eta'grad), Weight Update3/1(eta'grad), Weight Update2/1(eta'grad), Weight Update1/1(eta'grad), Bias Update1/1(eta'grad)
  Constant1/1 -> Mult8/1
  Mult6/1 -> AddSub/2
  eta'w11/1 -> AddSub1/2
  Hyperbolic Tangent1/1(Out1) -> Out/1, Mult6/1, Mult6/2
  AddSub1/1 -> Mult7/1
  AddSub/1 -> Mult7/2
  eta'w21/1 -> AddSub1/1
  Weight Update5/1(w11) -> Mult4/1
  x3/1 -> Mult2/2, Weight Update3/2(xin1)
  x5/1 -> Mult4/2, Weight Update5/2(xin1)
  Weight Update6/1(w11) -> Mult5/1
  Weight Update4/1(w11) -> Mult3/1
  x2/1 -> Mult1/2, Weight Update2/2(xin1)
  Weight Update1/1(w11) -> Mult/1
  Weight Update2/1(w11) -> Mult1/1
  Weight Update3/1(w11) -> Mult2/1
  x1/1 -> Mult/2, Weight Update1/2(xin1)
  x4/1 -> Mult3/2, Weight Update4/2(xin1)
  Mult1/1 -> Sum/2
  Mult4/1 -> Sum/5
  x6/1 -> Mult5/2, Weight Update6/2(xin1)
  Mult3/1 -> Sum/4
  Mult5/1 -> Sum/6
  Mult/1 -> Sum/1
  Mult2/1 -> Sum/3

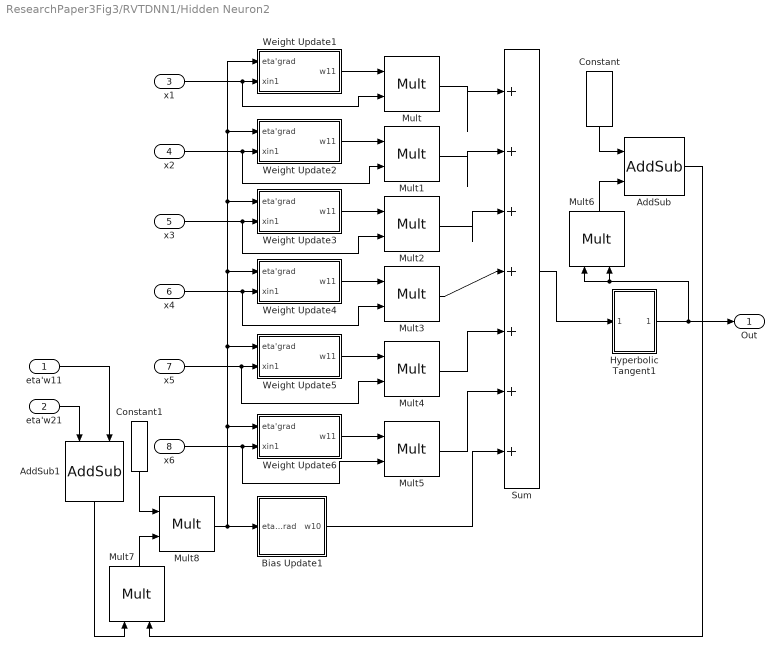
== system ResearchPaper3Fig3/RVTDNN1/Hidden Neuron2 ==
  eta'w11 : Inport
  eta'w21 : Inport  Port=2
  x1 : Inport  Port=3
  x2 : Inport  Port=4
  x3 : Inport  Port=5
  x4 : Inport  Port=6
  x5 : Inport  Port=7
  x6 : Inport  Port=8
  AddSub : xbsIndex_r4/AddSub  mode=Subtraction  use_carryin=off  use_carryout=off  en=off  latency=0  precision=Full  arith_type=Unsigned  n_bits=16  bin_pt=14  quantization=Truncate  overflow=Wrap  use_behavioral_HDL=off  hw_selection=Fabric  pipelined=off  dbl_ovrd=off  block_type=addsub
  AddSub1 : xbsIndex_r4/AddSub  mode=Addition  use_carryin=off  use_carryout=off  en=off  latency=0  precision=Full  arith_type=Unsigned  n_bits=16  bin_pt=14  quantization=Truncate  overflow=Wrap  use_behavioral_HDL=off  hw_selection=Fabric  pipelined=off  dbl_ovrd=off  block_type=addsub
  Bias Update1 : Subsystem
  Constant : xbsIndex_r4/Constant  const=1.0  gui_display_data_type=Fixed-point  arith_type=Signed (2's comp)  n_bits=16  bin_pt=14  preci_type=Single  exp_width=8  frac_width=24  explicit_period=off  period=1  equ=P=C  opselect=C  inp2=PCIN>>17  opr=+  inp1=P  carry=CIN  dbl_ovrd=off  block_type=constant
  Constant1 : xbsIndex_r4/Constant  const=0.1000000  gui_display_data_type=Fixed-point  arith_type=Signed (2's comp)  n_bits=32  bin_pt=24  preci_type=Single  exp_width=8  frac_width=24  explicit_period=off  period=1  equ=P=C  opselect=C  inp2=PCIN>>17  opr=+  inp1=P  carry=CIN  dbl_ovrd=off  block_type=constant
  Hyperbolic Tangent1 : Subsystem
  Mult{,1..8} (9 alike) : xbsIndex_r4/Mult  precision=Full  arith_type="Signed  (2's comp)"  n_bits=16  bin_pt=14  quantization=Truncate  overflow=Wrap  en=off  latency=0  use_behavioral_HDL=off  opt=Speed  use_embedded=on  optimum_pipeline=off  pipeline=on  dbl_ovrd=off  use_rpm=on  placement_style=Triangular  block_type=mult
  Sum : Sum  Inputs=|+++++++
  Weight Update1 : Subsystem
  Weight Update2 : Subsystem
  Weight Update3 : Subsystem
  Weight Update4 : Subsystem
  Weight Update5 : Subsystem
  Weight Update6 : Subsystem
  Out : Outport
  wires:
  Mult7/1 -> Mult8/2
  Sum/1 -> Hyperbolic Tangent1/1(In1)
  Bias Update1/1(w10) -> Sum/7
  Constant/1 -> AddSub/1
  Mult8/1 -> Weight Update6/1(eta'grad), Weight Update5/1(eta'grad), Weight Update4/1(eta'grad), Weight Update3/1(eta'grad), Weight Update2/1(eta'grad), Weight Update1/1(eta'grad), Bias Update1/1(eta'grad)
  Constant1/1 -> Mult8/1
  Mult6/1 -> AddSub/2
  eta'w11/1 -> AddSub1/2
  Hyperbolic Tangent1/1(Out1) -> Out/1, Mult6/1, Mult6/2
  AddSub1/1 -> Mult7/1
  AddSub/1 -> Mult7/2
  eta'w21/1 -> AddSub1/1
  Weight Update5/1(w11) -> Mult4/1
  x3/1 -> Mult2/2, Weight Update3/2(xin1)
  x5/1 -> Mult4/2, Weight Update5/2(xin1)
  Weight Update6/1(w11) -> Mult5/1
  Weight Update4/1(w11) -> Mult3/1
  x2/1 -> Mult1/2, Weight Update2/2(xin1)
  Weight Update1/1(w11) -> Mult/1
  Weight Update2/1(w11) -> Mult1/1
  Weight Update3/1(w11) -> Mult2/1
  x1/1 -> Mult/2, Weight Update1/2(xin1)
  x4/1 -> Mult3/2, Weight Update4/2(xin1)
  Mult1/1 -> Sum/2
  Mult4/1 -> Sum/5
  x6/1 -> Mult5/2, Weight Update6/2(xin1)
  Mult3/1 -> Sum/4
  Mult5/1 -> Sum/6
  Mult/1 -> Sum/1
  Mult2/1 -> Sum/3

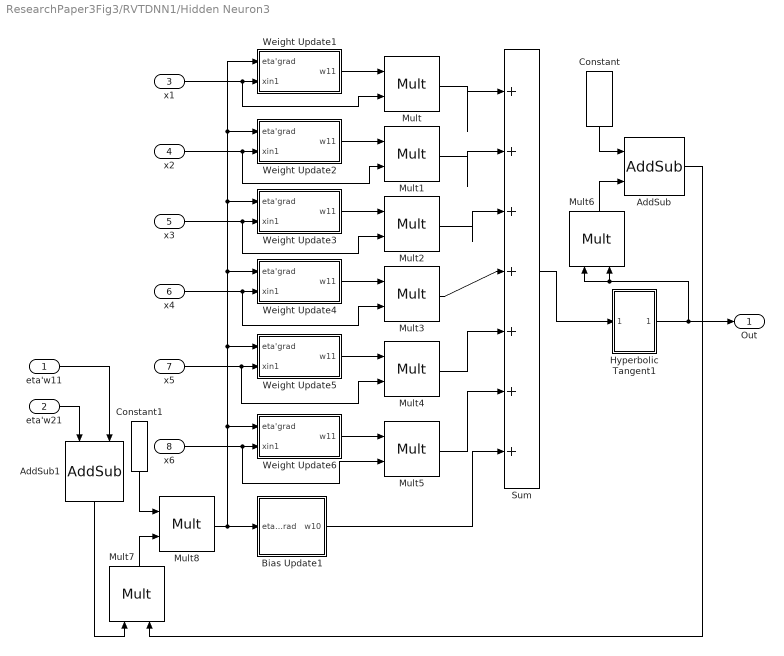
== system ResearchPaper3Fig3/RVTDNN1/Hidden Neuron3 ==
  eta'w11 : Inport
  eta'w21 : Inport  Port=2
  x1 : Inport  Port=3
  x2 : Inport  Port=4
  x3 : Inport  Port=5
  x4 : Inport  Port=6
  x5 : Inport  Port=7
  x6 : Inport  Port=8
  AddSub : xbsIndex_r4/AddSub  mode=Subtraction  use_carryin=off  use_carryout=off  en=off  latency=0  precision=Full  arith_type=Unsigned  n_bits=16  bin_pt=14  quantization=Truncate  overflow=Wrap  use_behavioral_HDL=off  hw_selection=Fabric  pipelined=off  dbl_ovrd=off  block_type=addsub
  AddSub1 : xbsIndex_r4/AddSub  mode=Addition  use_carryin=off  use_carryout=off  en=off  latency=0  precision=Full  arith_type=Unsigned  n_bits=16  bin_pt=14  quantization=Truncate  overflow=Wrap  use_behavioral_HDL=off  hw_selection=Fabric  pipelined=off  dbl_ovrd=off  block_type=addsub
  Bias Update1 : Subsystem
  Constant : xbsIndex_r4/Constant  const=1.0  gui_display_data_type=Fixed-point  arith_type=Signed (2's comp)  n_bits=16  bin_pt=14  preci_type=Single  exp_width=8  frac_width=24  explicit_period=off  period=1  equ=P=C  opselect=C  inp2=PCIN>>17  opr=+  inp1=P  carry=CIN  dbl_ovrd=off  block_type=constant
  Constant1 : xbsIndex_r4/Constant  const=0.1000000  gui_display_data_type=Fixed-point  arith_type=Signed (2's comp)  n_bits=32  bin_pt=24  preci_type=Single  exp_width=8  frac_width=24  explicit_period=off  period=1  equ=P=C  opselect=C  inp2=PCIN>>17  opr=+  inp1=P  carry=CIN  dbl_ovrd=off  block_type=constant
  Hyperbolic Tangent1 : Subsystem
  Mult{,1..8} (9 alike) : xbsIndex_r4/Mult  precision=Full  arith_type="Signed  (2's comp)"  n_bits=16  bin_pt=14  quantization=Truncate  overflow=Wrap  en=off  latency=0  use_behavioral_HDL=off  opt=Speed  use_embedded=on  optimum_pipeline=off  pipeline=on  dbl_ovrd=off  use_rpm=on  placement_style=Triangular  block_type=mult
  Sum : Sum  Inputs=|+++++++
  Weight Update1 : Subsystem
  Weight Update2 : Subsystem
  Weight Update3 : Subsystem
  Weight Update4 : Subsystem
  Weight Update5 : Subsystem
  Weight Update6 : Subsystem
  Out : Outport
  wires:
  Mult7/1 -> Mult8/2
  Sum/1 -> Hyperbolic Tangent1/1(In1)
  Bias Update1/1(w10) -> Sum/7
  Constant/1 -> AddSub/1
  Mult8/1 -> Weight Update6/1(eta'grad), Weight Update5/1(eta'grad), Weight Update4/1(eta'grad), Weight Update3/1(eta'grad), Weight Update2/1(eta'grad), Weight Update1/1(eta'grad), Bias Update1/1(eta'grad)
  Constant1/1 -> Mult8/1
  Mult6/1 -> AddSub/2
  eta'w11/1 -> AddSub1/2
  Hyperbolic Tangent1/1(Out1) -> Out/1, Mult6/1, Mult6/2
  AddSub1/1 -> Mult7/1
  AddSub/1 -> Mult7/2
  eta'w21/1 -> AddSub1/1
  Weight Update5/1(w11) -> Mult4/1
  x3/1 -> Mult2/2, Weight Update3/2(xin1)
  x5/1 -> Mult4/2, Weight Update5/2(xin1)
  Weight Update6/1(w11) -> Mult5/1
  Weight Update4/1(w11) -> Mult3/1
  x2/1 -> Mult1/2, Weight Update2/2(xin1)
  Weight Update1/1(w11) -> Mult/1
  Weight Update2/1(w11) -> Mult1/1
  Weight Update3/1(w11) -> Mult2/1
  x1/1 -> Mult/2, Weight Update1/2(xin1)
  x4/1 -> Mult3/2, Weight Update4/2(xin1)
  Mult1/1 -> Sum/2
  Mult4/1 -> Sum/5
  x6/1 -> Mult5/2, Weight Update6/2(xin1)
  Mult3/1 -> Sum/4
  Mult5/1 -> Sum/6
  Mult/1 -> Sum/1
  Mult2/1 -> Sum/3

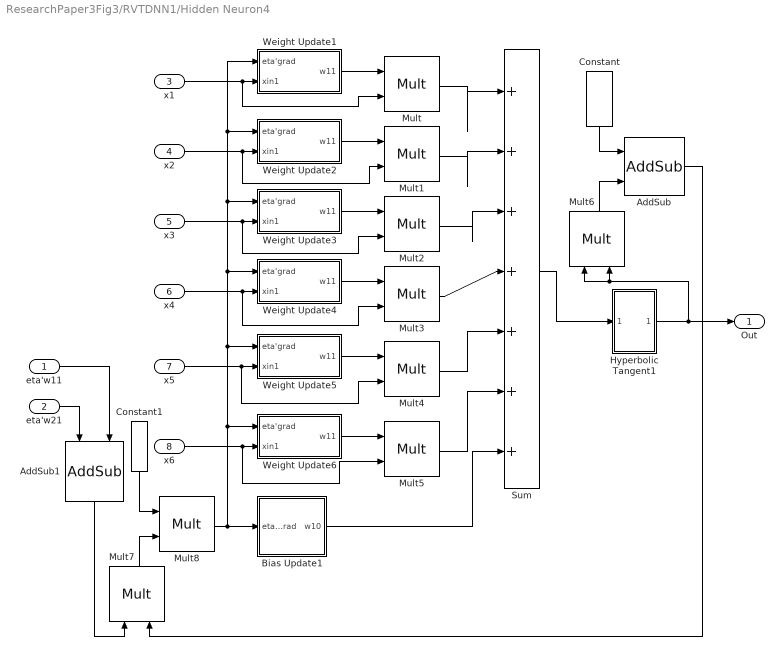
== system ResearchPaper3Fig3/RVTDNN1/Hidden Neuron4 ==
  eta'w11 : Inport
  eta'w21 : Inport  Port=2
  x1 : Inport  Port=3
  x2 : Inport  Port=4
  x3 : Inport  Port=5
  x4 : Inport  Port=6
  x5 : Inport  Port=7
  x6 : Inport  Port=8
  AddSub : xbsIndex_r4/AddSub  mode=Subtraction  use_carryin=off  use_carryout=off  en=off  latency=0  precision=Full  arith_type=Unsigned  n_bits=16  bin_pt=14  quantization=Truncate  overflow=Wrap  use_behavioral_HDL=off  hw_selection=Fabric  pipelined=off  dbl_ovrd=off  block_type=addsub
  AddSub1 : xbsIndex_r4/AddSub  mode=Addition  use_carryin=off  use_carryout=off  en=off  latency=0  precision=Full  arith_type=Unsigned  n_bits=16  bin_pt=14  quantization=Truncate  overflow=Wrap  use_behavioral_HDL=off  hw_selection=Fabric  pipelined=off  dbl_ovrd=off  block_type=addsub
  Bias Update1 : Subsystem
  Constant : xbsIndex_r4/Constant  const=1.0  gui_display_data_type=Fixed-point  arith_type=Signed (2's comp)  n_bits=16  bin_pt=14  preci_type=Single  exp_width=8  frac_width=24  explicit_period=off  period=1  equ=P=C  opselect=C  inp2=PCIN>>17  opr=+  inp1=P  carry=CIN  dbl_ovrd=off  block_type=constant
  Constant1 : xbsIndex_r4/Constant  const=0.1000000  gui_display_data_type=Fixed-point  arith_type=Signed (2's comp)  n_bits=32  bin_pt=24  preci_type=Single  exp_width=8  frac_width=24  explicit_period=off  period=1  equ=P=C  opselect=C  inp2=PCIN>>17  opr=+  inp1=P  carry=CIN  dbl_ovrd=off  block_type=constant
  Hyperbolic Tangent1 : Subsystem
  Mult{,1..8} (9 alike) : xbsIndex_r4/Mult  precision=Full  arith_type="Signed  (2's comp)"  n_bits=16  bin_pt=14  quantization=Truncate  overflow=Wrap  en=off  latency=0  use_behavioral_HDL=off  opt=Speed  use_embedded=on  optimum_pipeline=off  pipeline=on  dbl_ovrd=off  use_rpm=on  placement_style=Triangular  block_type=mult
  Sum : Sum  Inputs=|+++++++
  Weight Update1 : Subsystem
  Weight Update2 : Subsystem
  Weight Update3 : Subsystem
  Weight Update4 : Subsystem
  Weight Update5 : Subsystem
  Weight Update6 : Subsystem
  Out : Outport
  wires:
  Mult7/1 -> Mult8/2
  Sum/1 -> Hyperbolic Tangent1/1(In1)
  Bias Update1/1(w10) -> Sum/7
  Constant/1 -> AddSub/1
  Mult8/1 -> Weight Update6/1(eta'grad), Weight Update5/1(eta'grad), Weight Update4/1(eta'grad), Weight Update3/1(eta'grad), Weight Update2/1(eta'grad), Weight Update1/1(eta'grad), Bias Update1/1(eta'grad)
  Constant1/1 -> Mult8/1
  Mult6/1 -> AddSub/2
  eta'w11/1 -> AddSub1/2
  Hyperbolic Tangent1/1(Out1) -> Out/1, Mult6/1, Mult6/2
  AddSub1/1 -> Mult7/1
  AddSub/1 -> Mult7/2
  eta'w21/1 -> AddSub1/1
  Weight Update5/1(w11) -> Mult4/1
  x3/1 -> Mult2/2, Weight Update3/2(xin1)
  x5/1 -> Mult4/2, Weight Update5/2(xin1)
  Weight Update6/1(w11) -> Mult5/1
  Weight Update4/1(w11) -> Mult3/1
  x2/1 -> Mult1/2, Weight Update2/2(xin1)
  Weight Update1/1(w11) -> Mult/1
  Weight Update2/1(w11) -> Mult1/1
  Weight Update3/1(w11) -> Mult2/1
  x1/1 -> Mult/2, Weight Update1/2(xin1)
  x4/1 -> Mult3/2, Weight Update4/2(xin1)
  Mult1/1 -> Sum/2
  Mult4/1 -> Sum/5
  x6/1 -> Mult5/2, Weight Update6/2(xin1)
  Mult3/1 -> Sum/4
  Mult5/1 -> Sum/6
  Mult/1 -> Sum/1
  Mult2/1 -> Sum/3

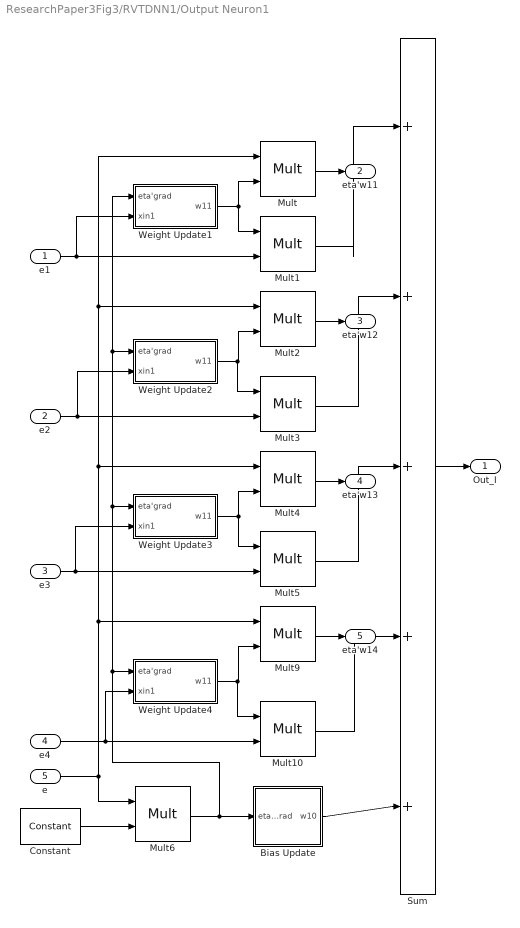
== system ResearchPaper3Fig3/RVTDNN1/Output Neuron1 ==
  e1 : Inport
  e2 : Inport  Port=2
  e3 : Inport  Port=3
  e4 : Inport  Port=4
  e : Inport  Port=5
  Bias Update : Subsystem
  Constant : xbsIndex_r4/Constant  const=16972656  gui_display_data_type=Fixed-point  arith_type=Signed (2's comp)  n_bits=64  bin_pt=14  preci_type=Single  exp_width=8  frac_width=24  explicit_period=off  period=1  equ=P=C  opselect=C  inp2=PCIN>>17  opr=+  inp1=P  carry=CIN  dbl_ovrd=off  block_type=constant
  Mult{,1..6,9..10} (9 alike) : xbsIndex_r4/Mult  precision=Full  arith_type="Signed  (2's comp)"  n_bits=16  bin_pt=14  quantization=Truncate  overflow=Wrap  en=off  latency=0  use_behavioral_HDL=off  opt=Speed  use_embedded=on  optimum_pipeline=off  pipeline=on  dbl_ovrd=off  use_rpm=on  placement_style=Triangular  block_type=mult
  Sum : Sum  Inputs=|+++++
  Weight Update1 : Subsystem
  Weight Update2 : Subsystem
  Weight Update3 : Subsystem
  Weight Update4 : Subsystem
  Out_I : Outport
  eta'w11 : Outport  Port=2
  eta'w12 : Outport  Port=3
  eta'w13 : Outport  Port=4
  eta'w14 : Outport  Port=5
  wires:
  e3/1 -> Weight Update3/2(xin1), Mult5/2
  e2/1 -> Weight Update2/2(xin1), Mult3/2
  e1/1 -> Weight Update1/2(xin1), Mult1/2
  e4/1 -> Weight Update4/2(xin1), Mult10/2
  Weight Update1/1(w11) -> Mult1/1, Mult/2
  Weight Update2/1(w11) -> Mult3/1, Mult2/2
  Weight Update3/1(w11) -> Mult5/1, Mult4/2
  Weight Update4/1(w11) -> Mult10/1, Mult9/2
  Mult/1 -> eta'w11/1
  Mult2/1 -> eta'w12/1
  Mult4/1 -> eta'w13/1
  Mult9/1 -> eta'w14/1
  Mult1/1 -> Sum/1
  Mult3/1 -> Sum/2
  Mult5/1 -> Sum/3
  Mult10/1 -> Sum/4
  Bias Update/1(w10) -> Sum/5
  Mult6/1 -> Weight Update4/1(eta'grad), Weight Update3/1(eta'grad), Weight Update2/1(eta'grad), Weight Update1/1(eta'grad), Bias Update/1(eta'grad)
  Constant/1 -> Mult6/2
  e/1 -> Mult4/1, Mult2/1, Mult/1, Mult9/1, Mult6/1
  Sum/1 -> Out_I/1
